simulink model "Buck_Model_eZdsp"  (R2020a)
settings: Solver=FixedStepDiscrete  StartTime=0.0  StopTime=5  FixedStep=T  RelTol=1e-3  EnableMultiTasking=on
undefined symbols (not defined in the file): C, ILmax, L, rL, T, Ubat, Ucmax
libraries: c280xlib x6, c2833xlib x2, simulink x2
settings Model: ExtModeTrigDuration=8  Creator=Nguyen Tung  LastModifiedBy=Nguyen Tung
settings OptimizationCC: DefaultUnderspecifiedDataType=single  StrengthReduction=on  PassReuseOutputArgsAs=Individual arguments  MaxStackSize=1024  OptimizeBlockOrder=speed  OptimizationPriority=Speed  OptimizationCustomize=off  MultiThreadedLoops=on  DenormalBehavior=FlushToZero  EfficientTunableParamExpr=on
settings DebuggingCC: ParameterTunabilityLossMsg=error
settings HardwareCC: ProdBitPerChar=16  ProdBitPerInt=16  ProdBitPerPointer=32  ProdBitPerSizeT=32  ProdBitPerPtrDiffT=32  ProdLargestAtomicInteger=Integer  ProdLargestAtomicFloat=None  ProdWordSize=16  ProdLongLongMode=on  ProdHWDeviceType=Texas Instruments->C2000
settings SFSimCC: MATLABDynamicMemAlloc=off
settings RTWCC: SystemTargetFile=ert.tlc  HardwareBoard=TI Delfino F2833x  TLCOptions=-aInlineSetEventsForThisBaseRateFcn=TLC_FALSE -aSuppressMultiTaskScheduler=TLC_FALSE -aRateBasedStepFcn=1  TemplateMakefile=ert_default_tmf  GenerateReport=on  Toolchain=Texas Instruments Code Composer Studio (C2000)
settings CodeAppCC: ForceParamTrailComments=on  IgnoreCustomStorageClasses=off  OperatorAnnotations=on  SimulinkDataObjDesc=on  SFDataObjDesc=on  InsertBlockDesc=on
settings ERTTargetCC: CodeReplacementLibrary=TI C28x  ExtModeStaticAllocSize=10000

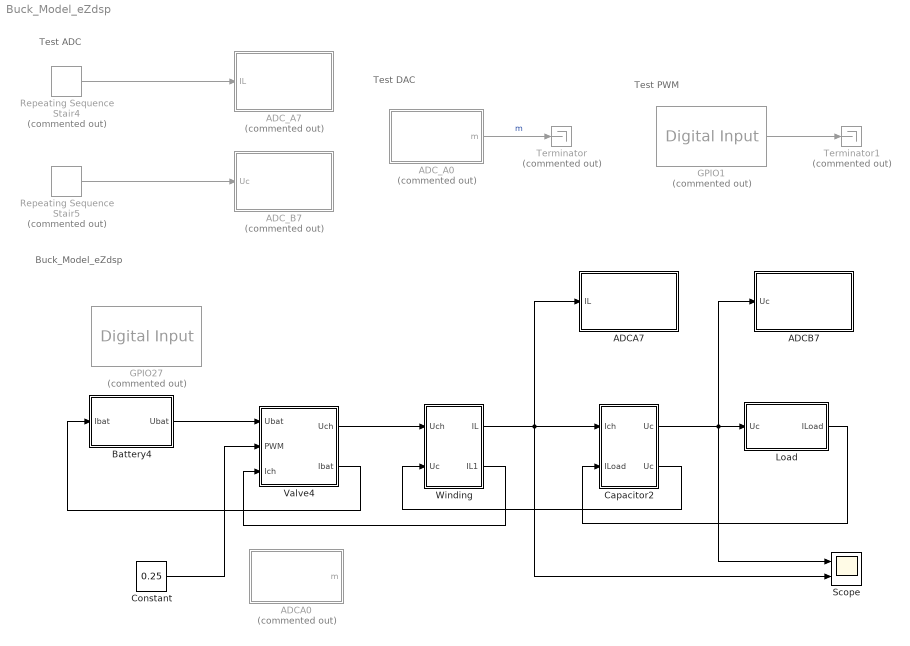
== system Buck_Model_eZdsp ==
  note: Test PWM
  note: Test DAC
  note: Test ADC
  note: Buck_Model_eZdsp
  ADCA0 : Subsystem  Commented=on
  ADCA7 : Subsystem
  ADCB7 : Subsystem
  ADC_A0 : Subsystem  Commented=on
  ADC_A7 : Subsystem  Commented=on
  ADC_B7 : Subsystem  Commented=on
  Battery4 : Subsystem  AncestorBlock=simulink/REM/SE
      mask Display:
      | plot(0,0,100,100, 1.2*[50,57.68,60.77,63.08,64.97,66.58,68,69.26,70.4, 	71.42,72.36,78.28,80,78.28,72.36,71.42,70.4, 	69.26,68,66.58,64.97,63.08,60.77,57.68,50,42.32, 	39.23,36.92,35.03,33.42,32,30.74,29.6,28.58, 	27.64,21.72,20,21.72,27.64,28.58,29.6,30.74,32, 	33.42,35.03,36.92,39.23,42.32,50]-10, 1.2*[20,21,22,23,24,25,26,27,28,29,30,40,50,60,70,71,72, 	73,74,75,76,77,78,79,80,79,78,77,76,75,74,73,72, 	71,70,60,50,40,30,29,28,27,26,25,24,23,22,21,20]-10)
      | disp('ES')
  Capacitor2 : Subsystem  AncestorBlock=simulink/REM/EA  mask(CM){}
      mask Display: plot(0,0,100,100,[10,10,90,90,10],[90,10,10,90,90], [10,90],[10,90])
  Constant : Constant  Value=0.25
  GPIO1 : c2833xlib/Digital Input  Commented=on  GPIO_Number=GPIO24~GPIO31  GPIO_Bit0=off  GPIO_Bit1=off  GPIO_Bit2=off  GPIO_Bit3=on  GPIO_Bit4=off  GPIO_Bit5=off  GPIO_Bit6=off  GPIO_Bit7=off  sampleTime=0.1  dataType=auto  GPIO_Bit0_Qualification=Sync to SYSCLKOUT  GPIO_Bit1_Qualification=Sync to SYSCLKOUT  GPIO_Bit2_Qualification=Sync to SYSCLKOUT  GPIO_Bit3_Qualification=Sync to SYSCLKOUT  GPIO_Bit4_Qualification=Sync to SYSCLKOUT  GPIO_Bit5_Qualification=Sync to SYSCLKOUT  GPIO_Bit6_Qualification=Sync to SYSCLKOUT  GPIO_Bit7_Qualification=Sync to SYSCLKOUT  Qualification_Period=-1
      settings: SourceProductBaseCode=TIC2000
  GPIO27 : c2833xlib/Digital Input  Commented=on  GPIO_Number=GPIO24~GPIO31  GPIO_Bit0=off  GPIO_Bit1=off  GPIO_Bit2=off  GPIO_Bit3=on  GPIO_Bit4=off  GPIO_Bit5=off  GPIO_Bit6=off  GPIO_Bit7=off  sampleTime=T  dataType=auto  GPIO_Bit0_Qualification=Sync to SYSCLKOUT  GPIO_Bit1_Qualification=Sync to SYSCLKOUT  GPIO_Bit2_Qualification=Sync to SYSCLKOUT  GPIO_Bit3_Qualification=Sync to SYSCLKOUT  GPIO_Bit4_Qualification=Sync to SYSCLKOUT  GPIO_Bit5_Qualification=Sync to SYSCLKOUT  GPIO_Bit6_Qualification=Sync to SYSCLKOUT  GPIO_Bit7_Qualification=Sync to SYSCLKOUT  Qualification_Period=-1
      settings: SourceProductBaseCode=TIC2000
  Load : Subsystem  AncestorBlock=simulink/REM/SE
      mask Display:
      | plot(0,0,100,100, 1.2*[50,57.68,60.77,63.08,64.97,66.58,68,69.26,70.4, 	71.42,72.36,78.28,80,78.28,72.36,71.42,70.4, 	69.26,68,66.58,64.97,63.08,60.77,57.68,50,42.32, 	39.23,36.92,35.03,33.42,32,30.74,29.6,28.58, 	27.64,21.72,20,21.72,27.64,28.58,29.6,30.74,32, 	33.42,35.03,36.92,39.23,42.32,50]-10, 1.2*[20,21,22,23,24,25,26,27,28,29,30,40,50,60,70,71,72, 	73,74,75,76,77,78,79,80,79,78,77,76,75,74,73,72, 	71,70,60,50,40,30,29,28,27,26,25,24,23,22,21,20]-10)
      | disp('MS')
  Repeating Sequence Stair4 : simulink/Sources/Repeating Sequence Stair  Commented=on  OutValues=[0 10 20 30 40 50 60].'  tsamp=T  OutMin=[]  OutMax=[]  OutDataTypeStr=double  OutputDataTypeScalingMode=double  OutDataType=fixdt(0,8)  ConRadixGroup=Best Precision: Vector-wise  OutScaling=2^-12
  Repeating Sequence Stair5 : simulink/Sources/Repeating Sequence Stair  Commented=on  OutValues=[0 50 100 150 200 250 300 350 400].'  tsamp=T  OutMin=[]  OutMax=[]  OutDataTypeStr=double  OutputDataTypeScalingMode=double  OutDataType=fixdt(0,8)  ConRadixGroup=Best Precision: Vector-wise  OutScaling=2^-12
  Scope : Scope  NumInputPorts=2
  Terminator : Terminator  Commented=on
  Terminator1 : Terminator  Commented=on
  Valve4 : Subsystem  AncestorBlock=simulink/REM/EC Elec  mask(Hacheur){}
      mask Display: plot(0,0,100,100,[10,10,90,90,10],[90,10,10,90,90])
  Winding : Subsystem  AncestorBlock=simulink/REM/EA  mask(CM){}
      mask Display: plot(0,0,100,100,[10,10,90,90,10],[90,10,10,90,90], [10,90],[10,90])
  wires:
  Capacitor2/2("Uc ") -> Winding/2(Uc)
  Valve4/1(Uch) -> Winding/1(Uch)
  Winding/1(IL) -> Scope/2, ADCA7/1(IL), Capacitor2/1(Ich)
  Load/1(ILoad) -> Capacitor2/2(ILoad)
  Battery4/1(Ubat) -> Valve4/1(Ubat)
  Capacitor2/1(Uc) -> Scope/1, ADCB7/1(Uc), Load/1(Uc)
  ADC_A0/1(m) -> Terminator/1  "m"
  GPIO1/1 -> Terminator1/1
  Repeating Sequence Stair4/1 -> ADC_A7/1(IL)
  Repeating Sequence Stair5/1 -> ADC_B7/1(Uc)
  Constant/1 -> Valve4/2(PWM)
  Valve4/2(Ibat) -> Battery4/1(Ibat)
  Winding/2(IL1) -> Valve4/3(Ich)

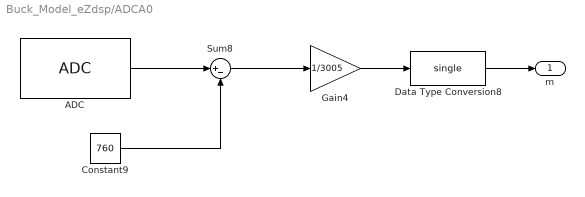
== system Buck_Model_eZdsp/ADCA0 ==
  ADC : c280xlib/ADC  useModule=A  useMode=Sequential  sourceSOC=Software  sourceSOC1=Software  sourceSOC2=ePWMxB  xint2_ADCSOC=31  Ts=T  dType=uint16  postInterrupt=off  numConversionsSingle=1  numConversionsDouble=1  conv0=ADCINA0  conv1=ADCINA1  conv2=ADCINA2  conv3=ADCINA3  conv4=ADCINA4  conv5=ADCINA5  conv6=ADCINA6  conv7=ADCINA7  conv8=ADCINB0  conv9=ADCINB1  conv10=ADCINB2  conv11=ADCINB3  conv12=ADCINB4  conv13=ADCINB5  conv14=ADCINB6  conv15=ADCINB7  convAB0=ADCINA0 and ADCINB0  convAB1=ADCINA1 and ADCINB1  convAB2=ADCINA2 and ADCINB2  convAB3=ADCINA3 and ADCINB3  convAB4=ADCINA4 and ADCINB4  convAB5=ADCINA5 and ADCINB5  convAB6=ADCINA6 and ADCINB6  convAB7=ADCINA7 and ADCINB7  convA0=ADCINA0  convA1=ADCINA1  convA2=ADCINA2  convA3=ADCINA3  convA4=ADCINA4  convA5=ADCINA5  convA6=ADCINA6  convA7=ADCINA7  convB0=ADCINB0  convB1=ADCINB1  convB2=ADCINB2  convB3=ADCINB3  convB4=ADCINB4  convB5=ADCINB5  convB6=ADCINB6  convB7=ADCINB7  c28xmultiPort=off  endma=off  chdma=1
      settings: SourceProductBaseCode=TIC2000
  Constant9 : Constant  Value=760
  Data Type Conversion8 : DataTypeConversion  OutMin=[0]  OutMax=[1]  OutDataTypeStr=single  SaturateOnIntegerOverflow=on
  Gain4 : Gain  Gain=1/3005
  Sum8 : Sum  Inputs=|+-
  m : Outport
  wires:
  Sum8/1 -> Gain4/1
  Constant9/1 -> Sum8/2
  ADC/1 -> Sum8/1
  Gain4/1 -> Data Type Conversion8/1
  Data Type Conversion8/1 -> m/1

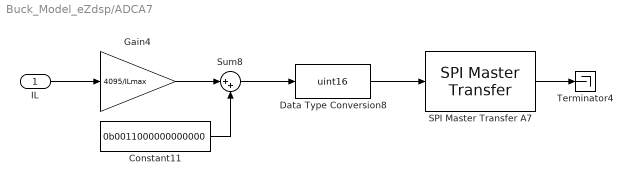
== system Buck_Model_eZdsp/ADCA7 ==
  IL : Inport
  Constant11 : Constant  Value=0b0011000000000000
  Data Type Conversion8 : DataTypeConversion  OutDataTypeStr=uint16
  Gain4 : Gain  Gain=4095/ILmax
  SPI Master Transfer A7 : c280xlib/SPI Master Transfer  SPISelect=SPI_A  ClockPolarity=Falling_edge  ClockPhase=No_delay  SPIModule=uint32(0)  Mode=Master  BusSpeed=uint32(1000000)  FirstBitToTransfer=Most significant bit (MSB)  ClockMode=0  BlockFunction=Transfer  EnableRegisterAddress=off  RegisterAddress=0  OutputDataType=int8  OutputDataLength=1  DataBits=16  UseCustomSSPin=Explicit GPIO calls  ActiveLowSSPin=Active low  Pin=7
      settings: SourceProductBaseCode=TIC2000
  Sum8 : Sum  Inputs=|++
  Terminator4 : Terminator
  wires:
  Gain4/1 -> Sum8/1
  Constant11/1 -> Sum8/2
  Data Type Conversion8/1 -> SPI Master Transfer A7/1
  Sum8/1 -> Data Type Conversion8/1
  SPI Master Transfer A7/1 -> Terminator4/1
  IL/1 -> Gain4/1

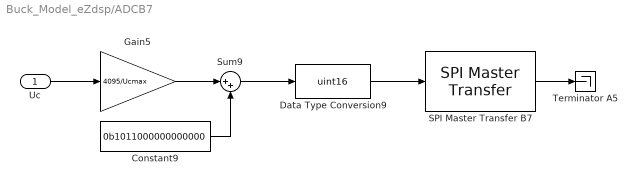
== system Buck_Model_eZdsp/ADCB7 ==
  Uc : Inport
  Constant9 : Constant  Value=0b1011000000000000
  Data Type Conversion9 : DataTypeConversion  OutDataTypeStr=uint16
  Gain5 : Gain  Gain=4095/Ucmax
  SPI Master Transfer B7 : c280xlib/SPI Master Transfer  SPISelect=SPI_A  ClockPolarity=Falling_edge  ClockPhase=No_delay  SPIModule=uint32(0)  Mode=Master  BusSpeed=uint32(1000000)  FirstBitToTransfer=Most significant bit (MSB)  ClockMode=0  BlockFunction=Transfer  EnableRegisterAddress=off  RegisterAddress=0  OutputDataType=int8  OutputDataLength=1  DataBits=16  UseCustomSSPin=Explicit GPIO calls  ActiveLowSSPin=Active low  Pin=7
      settings: SourceProductBaseCode=TIC2000
  Sum9 : Sum  Inputs=|++
  Terminator A5 : Terminator
  wires:
  Constant9/1 -> Sum9/2
  Gain5/1 -> Sum9/1
  SPI Master Transfer B7/1 -> Terminator A5/1
  Sum9/1 -> Data Type Conversion9/1
  Data Type Conversion9/1 -> SPI Master Transfer B7/1
  Uc/1 -> Gain5/1

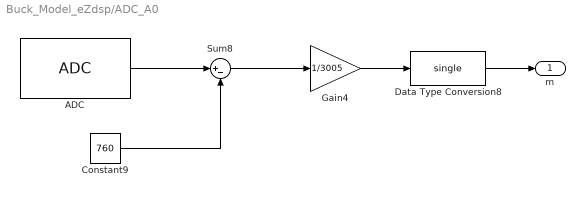
== system Buck_Model_eZdsp/ADC_A0 ==
  ADC : c280xlib/ADC  useModule=A  useMode=Sequential  sourceSOC=Software  sourceSOC1=Software  sourceSOC2=ePWMxB  xint2_ADCSOC=31  Ts=T  dType=uint16  postInterrupt=off  numConversionsSingle=1  numConversionsDouble=1  conv0=ADCINA0  conv1=ADCINA1  conv2=ADCINA2  conv3=ADCINA3  conv4=ADCINA4  conv5=ADCINA5  conv6=ADCINA6  conv7=ADCINA7  conv8=ADCINB0  conv9=ADCINB1  conv10=ADCINB2  conv11=ADCINB3  conv12=ADCINB4  conv13=ADCINB5  conv14=ADCINB6  conv15=ADCINB7  convAB0=ADCINA0 and ADCINB0  convAB1=ADCINA1 and ADCINB1  convAB2=ADCINA2 and ADCINB2  convAB3=ADCINA3 and ADCINB3  convAB4=ADCINA4 and ADCINB4  convAB5=ADCINA5 and ADCINB5  convAB6=ADCINA6 and ADCINB6  convAB7=ADCINA7 and ADCINB7  convA0=ADCINA0  convA1=ADCINA1  convA2=ADCINA2  convA3=ADCINA3  convA4=ADCINA4  convA5=ADCINA5  convA6=ADCINA6  convA7=ADCINA7  convB0=ADCINB0  convB1=ADCINB1  convB2=ADCINB2  convB3=ADCINB3  convB4=ADCINB4  convB5=ADCINB5  convB6=ADCINB6  convB7=ADCINB7  c28xmultiPort=off  endma=off  chdma=1
      settings: SourceProductBaseCode=TIC2000
  Constant9 : Constant  Value=760
  Data Type Conversion8 : DataTypeConversion  OutMin=[0]  OutMax=[1]  OutDataTypeStr=single  SaturateOnIntegerOverflow=on
  Gain4 : Gain  Gain=1/3005
  Sum8 : Sum  Inputs=|+-
  m : Outport
  wires:
  Sum8/1 -> Gain4/1
  Constant9/1 -> Sum8/2
  ADC/1 -> Sum8/1
  Gain4/1 -> Data Type Conversion8/1
  Data Type Conversion8/1 -> m/1

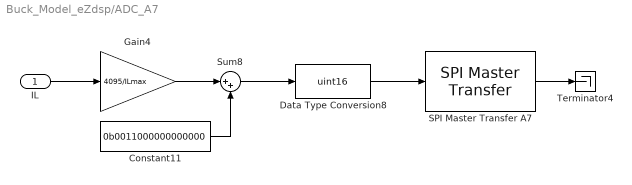
== system Buck_Model_eZdsp/ADC_A7 ==
  IL : Inport
  Constant11 : Constant  Value=0b0011000000000000
  Data Type Conversion8 : DataTypeConversion  OutDataTypeStr=uint16
  Gain4 : Gain  Gain=4095/ILmax
  SPI Master Transfer A7 : c280xlib/SPI Master Transfer  SPISelect=SPI_A  ClockPolarity=Falling_edge  ClockPhase=No_delay  SPIModule=uint32(0)  Mode=Master  BusSpeed=uint32(1000000)  FirstBitToTransfer=Most significant bit (MSB)  ClockMode=0  BlockFunction=Transfer  EnableRegisterAddress=off  RegisterAddress=0  OutputDataType=int8  OutputDataLength=1  DataBits=16  UseCustomSSPin=Explicit GPIO calls  ActiveLowSSPin=Active low  Pin=7
      settings: SourceProductBaseCode=TIC2000
  Sum8 : Sum  Inputs=|++
  Terminator4 : Terminator
  wires:
  Gain4/1 -> Sum8/1
  Constant11/1 -> Sum8/2
  Data Type Conversion8/1 -> SPI Master Transfer A7/1
  Sum8/1 -> Data Type Conversion8/1
  SPI Master Transfer A7/1 -> Terminator4/1
  IL/1 -> Gain4/1

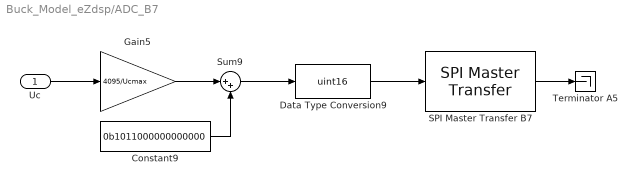
== system Buck_Model_eZdsp/ADC_B7 ==
  Uc : Inport
  Constant9 : Constant  Value=0b1011000000000000
  Data Type Conversion9 : DataTypeConversion  OutDataTypeStr=uint16
  Gain5 : Gain  Gain=4095/Ucmax
  SPI Master Transfer B7 : c280xlib/SPI Master Transfer  SPISelect=SPI_A  ClockPolarity=Falling_edge  ClockPhase=No_delay  SPIModule=uint32(0)  Mode=Master  BusSpeed=uint32(1000000)  FirstBitToTransfer=Most significant bit (MSB)  ClockMode=0  BlockFunction=Transfer  EnableRegisterAddress=off  RegisterAddress=0  OutputDataType=int8  OutputDataLength=1  DataBits=16  UseCustomSSPin=Explicit GPIO calls  ActiveLowSSPin=Active low  Pin=7
      settings: SourceProductBaseCode=TIC2000
  Sum9 : Sum  Inputs=|++
  Terminator A5 : Terminator
  wires:
  Constant9/1 -> Sum9/2
  Gain5/1 -> Sum9/1
  SPI Master Transfer B7/1 -> Terminator A5/1
  Sum9/1 -> Data Type Conversion9/1
  Data Type Conversion9/1 -> SPI Master Transfer B7/1
  Uc/1 -> Gain5/1

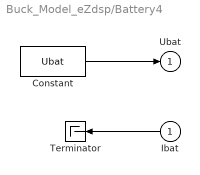
== system Buck_Model_eZdsp/Battery4 ==
  Ibat : Inport
  Constant : Constant  Value=Ubat  SampleTime=T
  Terminator : Terminator
  Ubat : Outport  InitialOutput=0  VectorParamsAs1DForOutWhenUnconnected=off
  wires:
  Constant/1 -> Ubat/1
  Ibat/1 -> Terminator/1

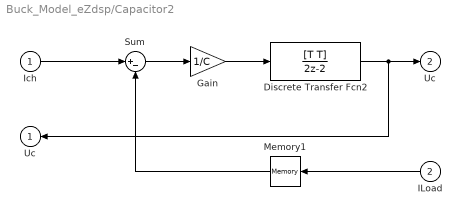
== system Buck_Model_eZdsp/Capacitor2 ==
  Ich : Inport
  ILoad : Inport  Port=2
  Discrete Transfer Fcn2 : DiscreteTransferFcn  Numerator=[T T]  Denominator=[2 -2]
  Gain : Gain  Gain=1/C
  Memory1 : Memory
  Sum : Sum  Inputs=|+-
  Uc : Outport  InitialOutput=0  VectorParamsAs1DForOutWhenUnconnected=off
  "Uc " : Outport  Port=2  InitialOutput=0  VectorParamsAs1DForOutWhenUnconnected=off
  wires:
  Ich/1 -> Sum/1
  Sum/1 -> Gain/1
  Gain/1 -> Discrete Transfer Fcn2/1
  ILoad/1 -> Memory1/1
  Discrete Transfer Fcn2/1 -> Uc/1, "Uc "/1
  Memory1/1 -> Sum/2

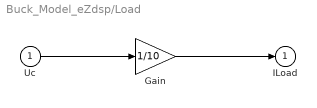
== system Buck_Model_eZdsp/Load ==
  Uc : Inport
  Gain : Gain  Gain=1/10
  ILoad : Outport  InitialOutput=0  VectorParamsAs1DForOutWhenUnconnected=off
  wires:
  Uc/1 -> Gain/1
  Gain/1 -> ILoad/1

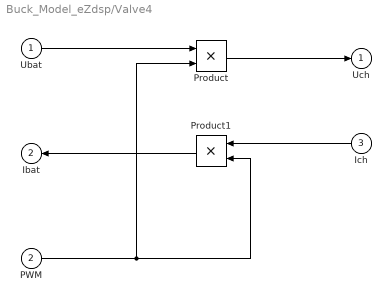
== system Buck_Model_eZdsp/Valve4 ==
  Ubat : Inport
  PWM : Inport  Port=2
  Ich : Inport  Port=3
  Product : Product
  Product1 : Product
  Uch : Outport  InitialOutput=0  VectorParamsAs1DForOutWhenUnconnected=off
  Ibat : Outport  Port=2  InitialOutput=0  VectorParamsAs1DForOutWhenUnconnected=off
  wires:
  Product/1 -> Uch/1
  Ubat/1 -> Product/1
  PWM/1 -> Product1/2, Product/2
  Product1/1 -> Ibat/1
  Ich/1 -> Product1/1

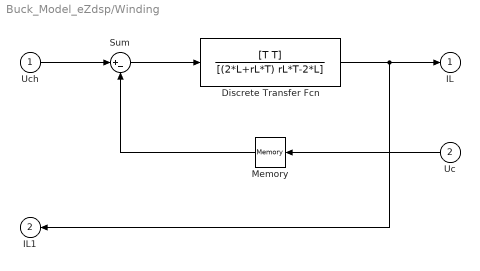
== system Buck_Model_eZdsp/Winding ==
  Uch : Inport
  Uc : Inport  Port=2
  Discrete Transfer Fcn : DiscreteTransferFcn  Numerator=[T T]  Denominator=[(2*L+rL*T) rL*T-2*L]
  Memory : Memory
  Sum : Sum  Inputs=|+-
  IL : Outport  InitialOutput=0  VectorParamsAs1DForOutWhenUnconnected=off
  IL1 : Outport  Port=2  InitialOutput=0  VectorParamsAs1DForOutWhenUnconnected=off
  wires:
  Uch/1 -> Sum/1
  Sum/1 -> Discrete Transfer Fcn/1
  Uc/1 -> Memory/1
  Discrete Transfer Fcn/1 -> IL1/1, IL/1
  Memory/1 -> Sum/2
